simulink model "lab4"  (R2023a)
settings: Solver=VariableStepAuto  StartTime=0.0  StopTime=3  RelTol=1e-3
settings Model: Creator=diontep  LastModifiedBy=diontep

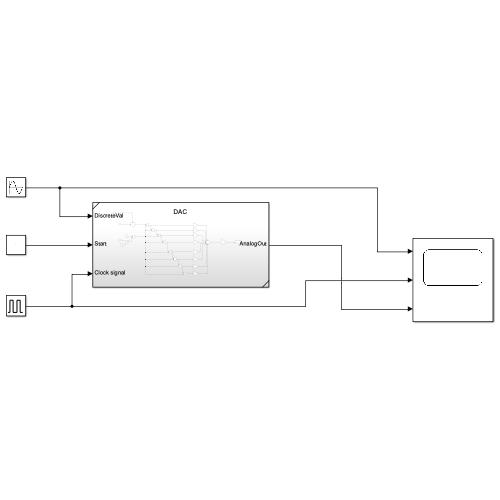
[thumbnail: Simulink's stored preview of the top-level diagram]
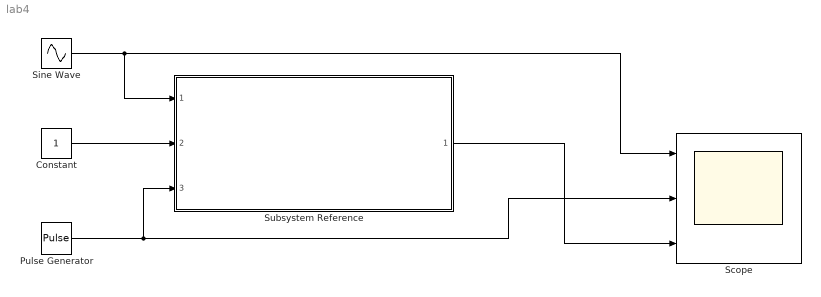
== system lab4 ==
  Constant : Constant
  Pulse Generator : DiscretePulseGenerator  PulseType=Time based  Period=0.1  PulseWidth=50
  Scope : Scope  NumInputPorts=3
  Sine Wave : Sin  Amplitude=128  SampleTime=0
  Subsystem Reference : Subsystem  ReferencedSubsystem=DAC
  wires:
  Sine Wave/1 -> Scope/1, Subsystem Reference/1
  Subsystem Reference/1 -> Scope/3
  Constant/1 -> Subsystem Reference/2
  Pulse Generator/1 -> Scope/2, Subsystem Reference/3
